simulink model "Project_2_Simulink_Code"  (R2021a)
settings: Solver=ode1  StartTime=0.0  StopTime=100  FixedStep=Ts  MaxStep=0.001  RelTol=1e-3  EnableMultiTasking=on
undefined symbols (not defined in the file): Kd, Ki, Kp, Ts
libraries: arduinolib x9
settings Model: SILPILModeSetting=veronly  ExtModeTrigDuration=2  Creator=arpit  LastModifiedBy=arpit
settings DataIOCC: ReturnWorkspaceOutputs=off
settings OptimizationCC: EnhancedBackFolding=on  PassReuseOutputArgsAs=Individual arguments  ZeroExternalMemoryAtStartup=off  ZeroInternalMemoryAtStartup=off  MaxStackSize=64  OptimizeBlockOrder=speed  DifferentSizesBufferReuse=on  EfficientTunableParamExpr=on
settings DebuggingCC: ParameterTunabilityLossMsg=error
settings HardwareCC: ProdBitPerPointer=32  ProdBitPerSizeT=32  ProdBitPerPtrDiffT=32  ProdLargestAtomicInteger=Long  ProdLargestAtomicFloat=Double  ProdWordSize=32  ProdHWDeviceType=ARM Compatible->ARM Cortex  UseEmbeddedCoderFeatures=off  UseSimulinkCoderFeatures=off
settings SFSimCC: MATLABDynamicMemAlloc=off
settings RTWCC: SystemTargetFile=ert.tlc  HardwareBoard=Arduino Due  TemplateMakefile=ert_default_tmf  Toolchain=Arduino ARM  BuildConfiguration=Faster Runs
settings CodeAppCC: ForceParamTrailComments=on  IgnoreCustomStorageClasses=off  OperatorAnnotations=on  SimulinkDataObjDesc=on  SFDataObjDesc=on  InsertBlockDesc=on
settings ERTTargetCC: SupportContinuousTime=on  SupportNonInlinedSFcns=on  SupportVariableSizeSignals=on  ExtModeTransport=3  ExtModeStaticAlloc=on  ExtModeStaticAllocSize=24576  ExtModeMexFile=ext_xcp  ExtModeIntrfLevel=Level2 - Open

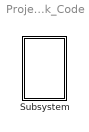
== system Project_2_Simulink_Code ==
  Subsystem : Subsystem

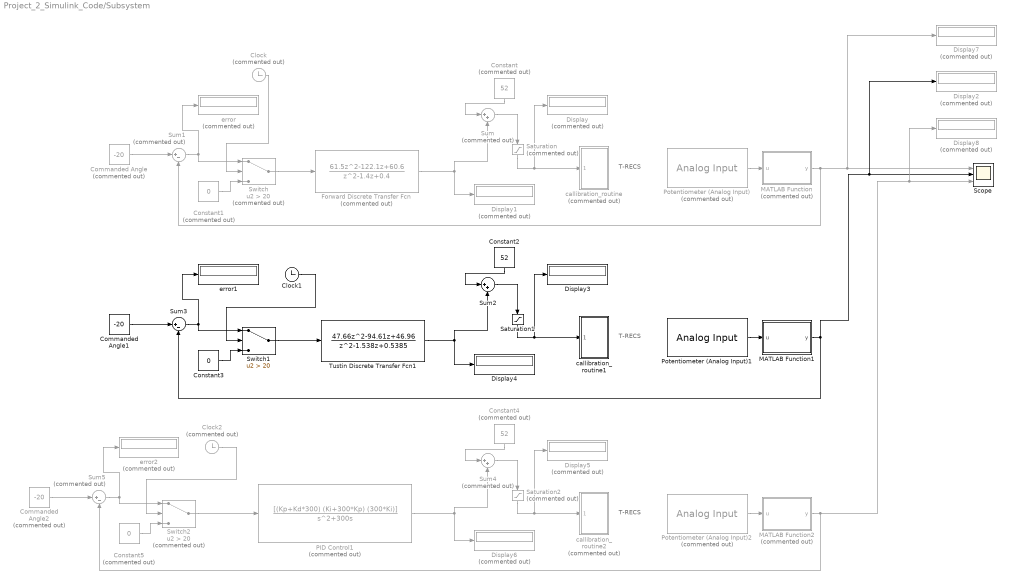
== system Project_2_Simulink_Code/Subsystem ==
  note: T-RECS
  note: T-RECS
  note: T-RECS
  Clock : Clock  Commented=on
  Clock1 : Clock
  Clock2 : Clock  Commented=on
  Commanded Angle : Constant  Commented=on  Value=-20  SampleTime=Ts
  Commanded Angle1 : Constant  Value=-20  SampleTime=Ts
  Commanded Angle2 : Constant  Commented=on  Value=-20  SampleTime=Ts
  Constant : Constant  Commented=on  Value=52  SampleTime=Ts
  Constant1 : Constant  Commented=on  Value=0
  Constant2 : Constant  Value=52  SampleTime=Ts
  Constant3 : Constant  Value=0
  Constant4 : Constant  Commented=on  Value=52  SampleTime=Ts
  Constant5 : Constant  Commented=on  Value=0
  Display{,1..2,5..8} (7 alike) : Display  Commented=on
  Display3 : Display
  Display4 : Display
  Forward Discrete Transfer Fcn : DiscreteTransferFcn  Commented=on  Numerator=[61.5 -122.1 60.6]  Denominator=[1 -1.4 0.4]  SampleTime=Ts
  MATLAB Function : MATLAB Function  Commented=on  TreatAsAtomicUnit=on
  MATLAB Function1 : MATLAB Function  TreatAsAtomicUnit=on
  MATLAB Function2 : MATLAB Function  Commented=on  TreatAsAtomicUnit=on
  PID Control1 : TransferFcn  Commented=on  Numerator=[(Kp+Kd*300) (Ki+300*Kp) (300*Ki)]  Denominator=[1 300 0]
  Potentiometer (Analog Input) : arduinolib/Analog Input  Commented=on  pinNumber=0  ReadResultsOnly=off  ConversionTriggerSource=Software  ExternalTriggerType=uint32( 0 )  OutputDataType=uint16  EnableConversionCompleteNotify=off  EnableOuputStatus=off  SampleTime=-1  blockPlatform=arduino
  Potentiometer (Analog Input)1 : arduinolib/Analog Input  pinNumber=0  ReadResultsOnly=off  ConversionTriggerSource=Software  ExternalTriggerType=uint32( 0 )  OutputDataType=uint16  EnableConversionCompleteNotify=off  EnableOuputStatus=off  SampleTime=-1  blockPlatform=arduino
  Potentiometer (Analog Input)2 : arduinolib/Analog Input  Commented=on  pinNumber=0  ReadResultsOnly=off  ConversionTriggerSource=Software  ExternalTriggerType=uint32( 0 )  OutputDataType=uint16  EnableConversionCompleteNotify=off  EnableOuputStatus=off  SampleTime=-1  blockPlatform=arduino
  Saturation : Saturate  Commented=on  UpperLimit=73.31  LowerLimit=44.2241
  Saturation1 : Saturate  UpperLimit=73.31  LowerLimit=44.2241
  Saturation2 : Saturate  Commented=on  UpperLimit=73.31  LowerLimit=44.2241
  Scope : Scope  NumInputPorts=3
  Sum : Sum  Commented=on  Inputs=|++
  Sum1 : Sum  Commented=on  Inputs=|+-
  Sum2 : Sum  Inputs=|++
  Sum3 : Sum  Inputs=|+-
  Sum4 : Sum  Commented=on  Inputs=|++
  Sum5 : Sum  Commented=on  Inputs=|+-
  Switch : Switch  Commented=on  Criteria=u2 > Threshold  Threshold=20
  Switch1 : Switch  Criteria=u2 > Threshold  Threshold=20
  Switch2 : Switch  Commented=on  Criteria=u2 > Threshold  Threshold=20
  Tustin Discrete Transfer Fcn1 : DiscreteTransferFcn  Numerator=[47.66 -94.61 46.96]  Denominator=[1 -1.538 0.5385]  SampleTime=Ts
  callibration_routine : Subsystem  Commented=on
  callibration_routine1 : Subsystem
  callibration_routine2 : Subsystem  Commented=on
  error : Display  Commented=on
  error1 : Display
  error2 : Display  Commented=on
  wires:
  Constant/1 -> Sum/1
  Sum/1 -> Saturation/1
  Commanded Angle/1 -> Sum1/1
  Potentiometer (Analog Input)/1 -> MATLAB Function/1(u)
  MATLAB Function/1(y) -> Sum1/2, Scope/1, Display7/1
  Saturation/1 -> callibration_routine/1(Control Input Angle (speed)), Display/1
  Sum1/1 -> Switch/1, error/1
  Forward Discrete Transfer Fcn/1 -> Sum/2, Display1/1
  Switch/1 -> Forward Discrete Transfer Fcn/1
  Constant1/1 -> Switch/3
  Clock/1 -> Switch/2
  Switch1/1 -> Tustin Discrete Transfer Fcn1/1
  Potentiometer (Analog Input)1/1 -> MATLAB Function1/1(u)
  Tustin Discrete Transfer Fcn1/1 -> Display4/1, Sum2/2
  Constant3/1 -> Switch1/3
  Clock1/1 -> Switch1/2
  MATLAB Function1/1(y) -> Scope/2, Display2/1, Sum3/2
  Saturation1/1 -> callibration_routine1/1(Control Input Angle (speed)), Display3/1
  Sum2/1 -> Saturation1/1
  Constant2/1 -> Sum2/1
  Commanded Angle1/1 -> Sum3/1
  Sum3/1 -> Switch1/1, error1/1
  Sum5/1 -> Switch2/1, error2/1
  Constant4/1 -> Sum4/1
  Commanded Angle2/1 -> Sum5/1
  Constant5/1 -> Switch2/3
  Sum4/1 -> Saturation2/1
  Saturation2/1 -> callibration_routine2/1(Control Input Angle (speed)), Display5/1
  MATLAB Function2/1(y) -> Display8/1, Scope/3, Sum5/2
  PID Control1/1 -> Display6/1, Sum4/2
  Potentiometer (Analog Input)2/1 -> MATLAB Function2/1(u)
  Clock2/1 -> Switch2/2
  Switch2/1 -> PID Control1/1

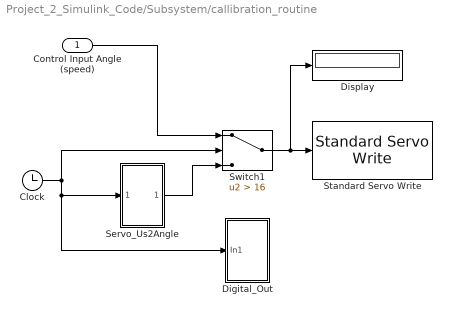
== system Project_2_Simulink_Code/Subsystem/callibration_routine ==
  Control Input Angle (speed) : Inport
  Clock : Clock
  Digital_Out : Subsystem
  Display : Display
  Servo_Us2Angle : Subsystem
  Standard Servo Write : arduinolib/Standard Servo Write  pinNumber=6  ServoIndex=0  blockPlatform=ARDUINO
  Switch1 : Switch  Criteria=u2 > Threshold  Threshold=16
  wires:
  Switch1/1 -> Display/1, Standard Servo Write/1
  Clock/1 -> Switch1/2, Digital_Out/1(In1), Servo_Us2Angle/1(In1)
  Servo_Us2Angle/1(Out1) -> Switch1/3
  Control Input Angle (speed)/1 -> Switch1/1

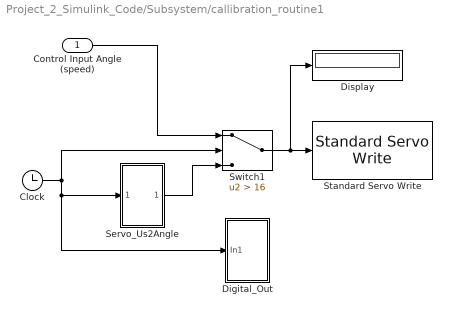
== system Project_2_Simulink_Code/Subsystem/callibration_routine1 ==
  Control Input Angle (speed) : Inport
  Clock : Clock
  Digital_Out : Subsystem
  Display : Display
  Servo_Us2Angle : Subsystem
  Standard Servo Write : arduinolib/Standard Servo Write  pinNumber=6  ServoIndex=0  blockPlatform=ARDUINO
  Switch1 : Switch  Criteria=u2 > Threshold  Threshold=16
  wires:
  Switch1/1 -> Display/1, Standard Servo Write/1
  Clock/1 -> Switch1/2, Digital_Out/1(In1), Servo_Us2Angle/1(In1)
  Servo_Us2Angle/1(Out1) -> Switch1/3
  Control Input Angle (speed)/1 -> Switch1/1

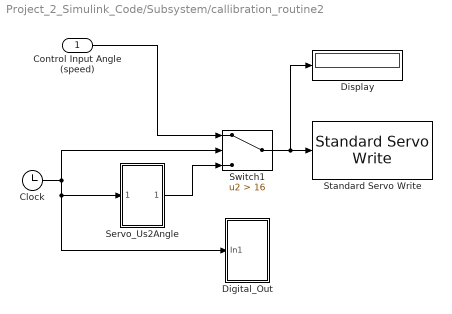
== system Project_2_Simulink_Code/Subsystem/callibration_routine2 ==
  Control Input Angle (speed) : Inport
  Clock : Clock
  Digital_Out : Subsystem
  Display : Display
  Servo_Us2Angle : Subsystem
  Standard Servo Write : arduinolib/Standard Servo Write  pinNumber=6  ServoIndex=0  blockPlatform=ARDUINO
  Switch1 : Switch  Criteria=u2 > Threshold  Threshold=16
  wires:
  Switch1/1 -> Display/1, Standard Servo Write/1
  Clock/1 -> Switch1/2, Digital_Out/1(In1), Servo_Us2Angle/1(In1)
  Servo_Us2Angle/1(Out1) -> Switch1/3
  Control Input Angle (speed)/1 -> Switch1/1

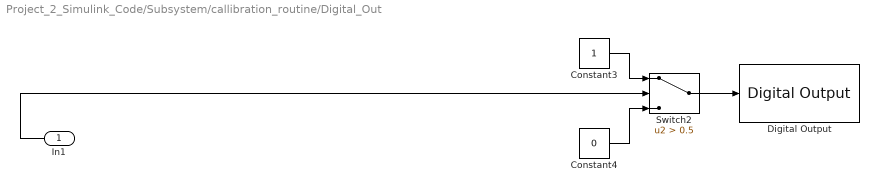
== system Project_2_Simulink_Code/Subsystem/callibration_routine/Digital_Out ==
  In1 : Inport
  Constant3 : Constant  SampleTime=Ts
  Constant4 : Constant  Value=0  SampleTime=Ts
  Digital Output : arduinolib/Digital Output  pinNumber=10  Direction=output  blockPlatform=arduino
  Switch2 : Switch  Criteria=u2 > Threshold  Threshold=0.5
  wires:
  Constant4/1 -> Switch2/3
  Switch2/1 -> Digital Output/1
  Constant3/1 -> Switch2/1
  In1/1 -> Switch2/2

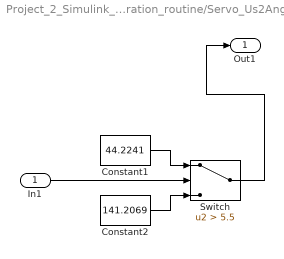
== system Project_2_Simulink_Code/Subsystem/callibration_routine/Servo_Us2Angle ==
  In1 : Inport
  Constant1 : Constant  Value=44.2241  SampleTime=Ts
  Constant2 : Constant  Value=141.2069  SampleTime=Ts
  Switch : Switch  Criteria=u2 > Threshold  Threshold=5.5
  Out1 : Outport
  wires:
  In1/1 -> Switch/2
  Constant1/1 -> Switch/1
  Constant2/1 -> Switch/3
  Switch/1 -> Out1/1

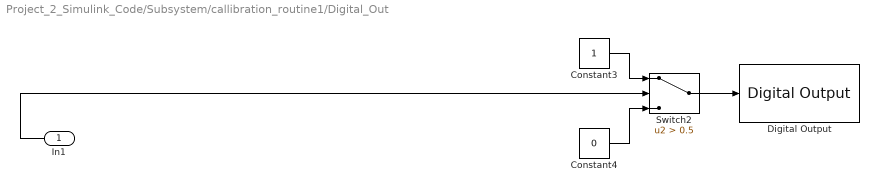
== system Project_2_Simulink_Code/Subsystem/callibration_routine1/Digital_Out ==
  In1 : Inport
  Constant3 : Constant  SampleTime=Ts
  Constant4 : Constant  Value=0  SampleTime=Ts
  Digital Output : arduinolib/Digital Output  pinNumber=10  Direction=output  blockPlatform=arduino
  Switch2 : Switch  Criteria=u2 > Threshold  Threshold=0.5
  wires:
  Constant4/1 -> Switch2/3
  Switch2/1 -> Digital Output/1
  Constant3/1 -> Switch2/1
  In1/1 -> Switch2/2

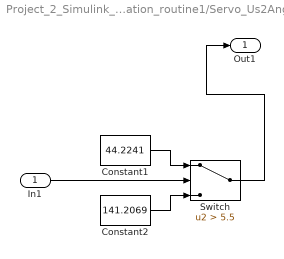
== system Project_2_Simulink_Code/Subsystem/callibration_routine1/Servo_Us2Angle ==
  In1 : Inport
  Constant1 : Constant  Value=44.2241  SampleTime=Ts
  Constant2 : Constant  Value=141.2069  SampleTime=Ts
  Switch : Switch  Criteria=u2 > Threshold  Threshold=5.5
  Out1 : Outport
  wires:
  In1/1 -> Switch/2
  Constant1/1 -> Switch/1
  Constant2/1 -> Switch/3
  Switch/1 -> Out1/1

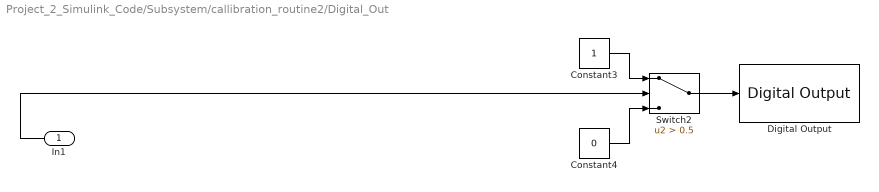
== system Project_2_Simulink_Code/Subsystem/callibration_routine2/Digital_Out ==
  In1 : Inport
  Constant3 : Constant  SampleTime=Ts
  Constant4 : Constant  Value=0  SampleTime=Ts
  Digital Output : arduinolib/Digital Output  pinNumber=10  Direction=output  blockPlatform=arduino
  Switch2 : Switch  Criteria=u2 > Threshold  Threshold=0.5
  wires:
  Constant4/1 -> Switch2/3
  Switch2/1 -> Digital Output/1
  Constant3/1 -> Switch2/1
  In1/1 -> Switch2/2

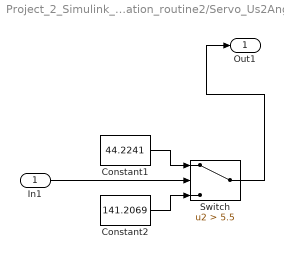
== system Project_2_Simulink_Code/Subsystem/callibration_routine2/Servo_Us2Angle ==
  In1 : Inport
  Constant1 : Constant  Value=44.2241  SampleTime=Ts
  Constant2 : Constant  Value=141.2069  SampleTime=Ts
  Switch : Switch  Criteria=u2 > Threshold  Threshold=5.5
  Out1 : Outport
  wires:
  In1/1 -> Switch/2
  Constant1/1 -> Switch/1
  Constant2/1 -> Switch/3
  Switch/1 -> Out1/1

== matlab function Project_2_Simulink_Code/Subsystem/MATLAB Function ==
  data: u input; y output
function y = fcn(u)

y = interp1([3940, 2300], [-39, 15], double(u));

== matlab function Project_2_Simulink_Code/Subsystem/MATLAB Function2 ==
  data: u input; y output
function y = fcn(u)

y = interp1([3940, 2300], [-39, 15], double(u));

== matlab function Project_2_Simulink_Code/Subsystem/MATLAB Function1 ==
  data: u input; y output
function y = fcn(u)

y = interp1([3940, 2300], [-39, 15], double(u));
